simulink model "sources"  (R2022a)
settings: Solver=VariableStepAuto  StartTime=0.0  StopTime=10.0  RelTol=1e-3
libraries: simulink x1
settings Model: Creator=Home computer  LastModifiedBy=Home computer

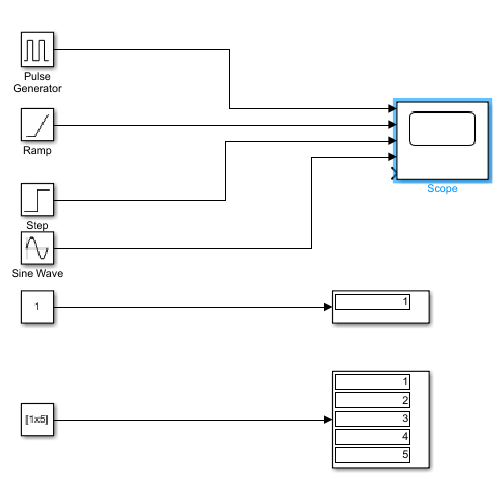
[thumbnail: Simulink's stored preview of the top-level diagram]
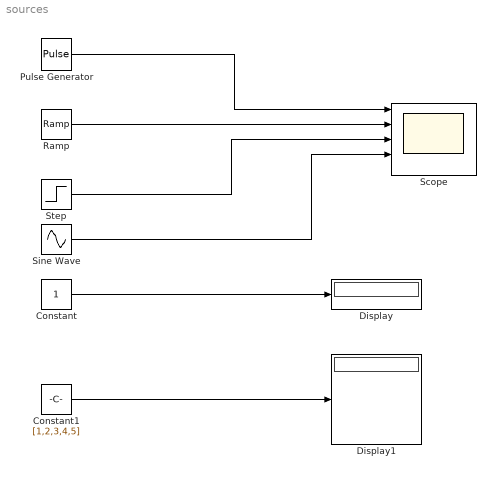
== system sources ==
  Constant : Constant
  Constant1 : Constant  Value=[1,2,3,4,5]
  Display : Display
  Display1 : Display
  Pulse Generator : DiscretePulseGenerator  PulseType=Time based  Amplitude=5  PulseWidth=10
  Ramp : simulink/Sources/Ramp  slope=2  start=5  InitialOutput=0
  Scope : Scope  NumInputPorts=5
  Sine Wave : Sin  Amplitude=3  SampleTime=0
  Step : Step  Time=2  After=10  SampleTime=0
  wires:
  Pulse Generator/1 -> Scope/1
  Ramp/1 -> Scope/2
  Step/1 -> Scope/3
  Sine Wave/1 -> Scope/4
  Constant/1 -> Display/1
  Constant1/1 -> Display1/1
